simulink model "half_car"  (R2020a)
settings: Solver=FixedStepAuto  StartTime=0.0  StopTime=1.5  FixedStep=0.0001  RelTol=1e-3
undefined symbols (not defined in the file or in its folder): A, B, C, K, M, tau
settings Model: Creator=User  LastModifiedBy=User

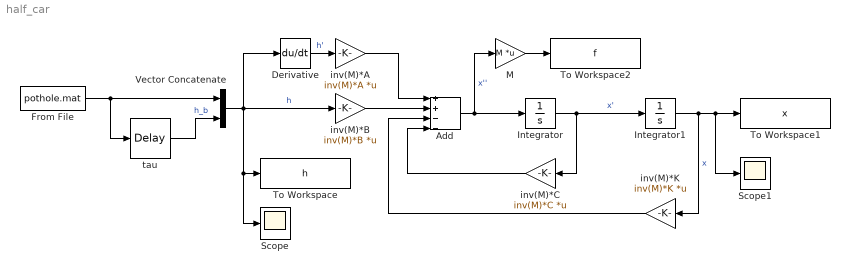
== system half_car ==
  Add : Sum  Inputs=++--
  Derivative : Derivative
  From File : FromFile  FileName=pothole.mat
  Integrator : Integrator
  Integrator1 : Integrator
  M : Gain  Gain=M  Multiplication=Matrix(K*u) (u vector)
  Scope : Scope
  Scope1 : Scope
  To Workspace : ToWorkspace  VariableName=h  SampleTime=-1
  To Workspace1 : ToWorkspace  VariableName=x  SampleTime=-1
  To Workspace2 : ToWorkspace  VariableName=f  SampleTime=-1
  Vector Concatenate : Concatenate
  inv(M)*A : Gain  Gain=inv(M)*A  Multiplication=Matrix(K*u) (u vector)
  inv(M)*B : Gain  Gain=inv(M)*B  Multiplication=Matrix(K*u) (u vector)
  inv(M)*C : Gain  Gain=inv(M)*C  Multiplication=Matrix(K*u) (u vector)
  inv(M)*K : Gain  Gain=inv(M)*K  Multiplication=Matrix(K*u) (u vector)
  tau : TransportDelay  DelayTime=tau
  wires:
  inv(M)*C/1 -> Add/4
  Add/1 -> M/1, Integrator/1  "x''"
  Integrator/1 -> inv(M)*C/1, Integrator1/1  "x'"
  Integrator1/1 -> Scope1/1, To Workspace1/1, inv(M)*K/1  "x"
  inv(M)*K/1 -> Add/3
  inv(M)*B/1 -> Add/2
  Derivative/1 -> inv(M)*A/1  "h'"
  inv(M)*A/1 -> Add/1
  tau/1 -> Vector Concatenate/2  "h_b"
  Vector Concatenate/1 -> To Workspace/1, Scope/1, Derivative/1, inv(M)*B/1  "h"
  From File/1 -> Vector Concatenate/1, tau/1
  M/1 -> To Workspace2/1
